simulink model "MSFartoystyring22old"  (Simulink 9.0)
settings: Solver=ode45  StartTime=tstart  StopTime=tstop  RelTol=1e-3  EnableMultiTasking=on
values from neighbouring files (symbols this model uses):
  c = 1    [run22.m]    (also in run23.m = norm(C))
  d1 = -0.0021    [init_controllers.m]
  d2 = 1.0377    [init_controllers.m]
  K = 0.0322    [init_controllers.m]    (also in run_task_1_2.m = x(2))
  Kd = 3*lambda_heading    (= 0.75)    [init_controllers.m]
  Ki = lambda_heading^3    (= 0.015625)    [init_controllers.m]
  Ki_guidance = 0.1    [run22.m]
  Ki_speed = lambda_speed^2    (= 0.09)    [init_controllers.m]
  Kp = 3*lambda_heading^2    (= 0.1875)    [init_controllers.m]
  Kp_guidance = 10    [run22.m]
  Kp_speed = 2*lambda_speed    (= 0.6)    [init_controllers.m]
  m = 5550    [init_controllers.m]
  omega_n = 0.008    [init_controllers.m]
  psi0 = 150*deg2rad    (= 2.61799387799)    [run22.m]    (also in run23.m = 0)
  r0 = 0    [run22.m]    (also in run23.m)
  T = 65.6949    [init_controllers.m]    (also in run_task_1_2.m = 1/x(1))
  tsamp = 10    [run22.m]    (also in run23.m)
  u_r_0 = 100    [init_controllers.m]
  v0 = [6.63 0]'    [run22.m]    (also in run23.m)
undefined symbols (not defined in the file or in its folder): guidance_control, msfartoystyring, WP, zeta
undefined symbols (not defined in the file): p0
settings Model: SuppressorTable=22 serialization::archive 11 0 6 0 0 0 0 0  Creator=christh  LastModifiedBy=henningward  ExtModeAutoUpdateStatusClock=off
settings DataIOCC: LimitDataPoints=on  SignalLoggingSaveFormat=ModelDataLogs
settings OptimizationCC: ExpressionDepthLimit=2147483647  InitFltsAndDblsToZero=on
settings DebuggingCC: SolverPrmCheckMsg=warning  FcnCallInpInsideContextMsg=warning  StateNameClashWarn=warning
settings GRTTargetCC: GeneratePreprocessorConditionals=Disable all  CombineOutputUpdateFcns=off  GRTInterface=on

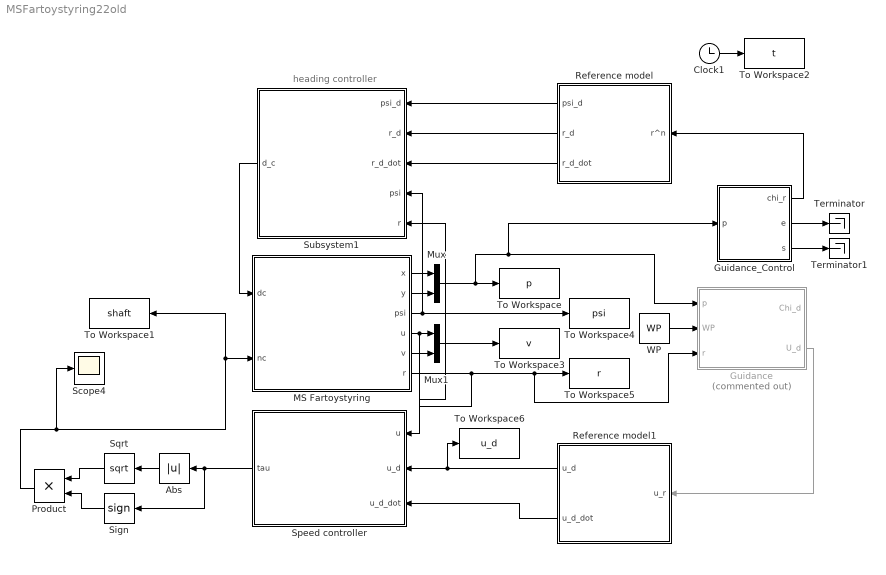
== system MSFartoystyring22old ==
  note: heading controller
  Abs : Abs
  Clock1 : Clock
  "Guidance " : Subsystem  Commented=on
  Guidance_Control : Subsystem
  MS Fartoystyring : Subsystem  mask(MS Fartoystyring for Assignment 3 G&C){x0=p0(1), y0=p0(2), u0=v0(1), v0=v0(2), psi0=psi0, r0=r0, c=c}
      mask prompts: x0 "x(t0) (m)"; y0 "y(t0) (m)"; u0 "u(t0) (m/s)"; v0 "v(t0) (m/s)"; psi0 "psi(t0) (rad)"; r0 "r(t0) (rad/s)"; c "current (0 or 1)"
      mask help:
      | Block corresponding to Figure 1 in the assignment text. Gives the response of the ship.
      |
      | The design speed of MS Fartoystyring is u=8.23 m/s.
      |
      | Input:
      | dc: commanded rudder (rad), dmax=25*pi/180
      | nc: commanded shaft speed (rad/s), nmax=85*2*pi/60
      |
      | Output:
      | x: north pos (m)
      | y: east pos (m)
      | u: surge (m/s)
      | v: sway (m/s)
      | psi: heading (rad)
      | r: yaw (rad/s)
      mask Help: Comments, bugs and help requests can be directed to the TA. Email on course website.
  Mux : Mux  Inputs=2
  Mux1 : Mux  Inputs=2
  Product : Product
  Reference model : Subsystem
  Reference model1 : Subsystem
  Scope4 : Scope
  Sign : Signum
  Speed controller : Subsystem
  Sqrt : Sqrt  SaturateOnIntegerOverflow=on
  Subsystem1 : Subsystem
  Terminator : Terminator
  Terminator1 : Terminator
  To Workspace : ToWorkspace  VariableName=p  SampleTime=tsamp
  To Workspace1 : ToWorkspace  VariableName=shaft  SampleTime=tsamp
  To Workspace2 : ToWorkspace  VariableName=t  SampleTime=tsamp
  To Workspace3 : ToWorkspace  VariableName=v  SampleTime=tsamp
  To Workspace4 : ToWorkspace  VariableName=psi  SampleTime=tsamp
  To Workspace5 : ToWorkspace  VariableName=r  SampleTime=tsamp
  To Workspace6 : ToWorkspace  VariableName=u_d  SampleTime=tsamp
  WP : Constant  Value=WP
  wires:
  MS Fartoystyring/1(x) -> Mux/1
  MS Fartoystyring/2(y) -> Mux/2
  MS Fartoystyring/4(u) -> Speed controller/1("u   "), Mux1/1
  MS Fartoystyring/5(v) -> Mux1/2
  Mux/1 -> Guidance_Control/1(p), "Guidance "/1(p), To Workspace/1
  Mux1/1 -> To Workspace3/1
  MS Fartoystyring/6(r) -> Subsystem1/5(r), "Guidance "/3(r), To Workspace5/1
  Subsystem1/1("d_c ") -> MS Fartoystyring/1(dc)
  Clock1/1 -> To Workspace2/1
  Speed controller/1("tau  ") -> Sign/1, Abs/1
  Abs/1 -> Sqrt/1
  Sign/1 -> Product/2
  Sqrt/1 -> Product/1
  Product/1 -> Scope4/1, To Workspace1/1, MS Fartoystyring/2(nc)
  Reference model/2(r_d) -> Subsystem1/2(r_d)
  Reference model/1(psi_d) -> Subsystem1/1(psi_d)
  Reference model/3(r_d_dot) -> Subsystem1/3(r_d_dot)
  MS Fartoystyring/3(psi) -> To Workspace4/1, Subsystem1/4("psi   ")
  Reference model1/1(u_d) -> To Workspace6/1, Speed controller/2(u_d)
  Reference model1/2(u_d_dot) -> Speed controller/3(u_d_dot)
  "Guidance "/2(U_d) -> Reference model1/1(u_r)
  WP/1 -> "Guidance "/2(WP)
  Guidance_Control/2(e) -> Terminator/1
  Guidance_Control/3(s) -> Terminator1/1
  Guidance_Control/1(chi_r) -> Reference model/1(r^n)

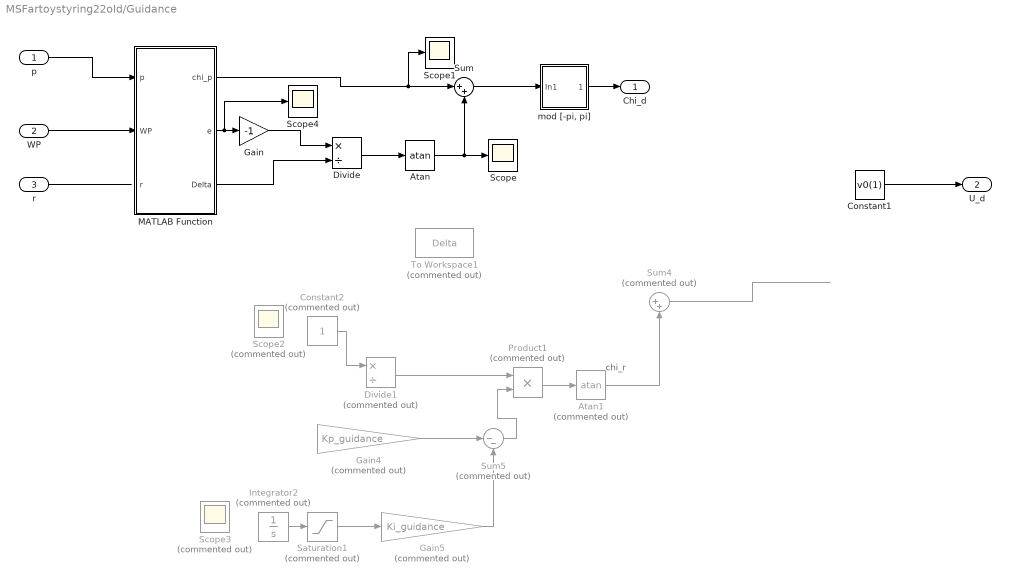
== system MSFartoystyring22old/Guidance  ==
  note: chi_r
  p : Inport
  WP : Inport  Port=2
  r : Inport  Port=3
  Atan : Trigonometry  Operator=atan
  Atan1 : Trigonometry  Commented=on  Operator=atan
  Constant1 : Constant  Value=v0(1)
  Constant2 : Constant  Commented=on
  Divide : Product  Inputs=*/
  Divide1 : Product  Commented=on  Inputs=*/
  Gain : Gain  Gain=-1
  Gain4 : Gain  Commented=on  Gain=Kp_guidance
  Gain5 : Gain  Commented=on  Gain=Ki_guidance
  Integrator2 : Integrator  Commented=on
  MATLAB Function : MATLAB Function  TreatAsAtomicUnit=on
  Product1 : Product  Commented=on
  Saturation1 : Saturate  Commented=on  UpperLimit=inf  LowerLimit=-inf
  Scope : Scope
  Scope1 : Scope
  Scope2 : Scope  Commented=on
  Scope3 : Scope  Commented=on
  Scope4 : Scope
  Sum : Sum  Inputs=|++
  Sum4 : Sum  Commented=on  Inputs=|++
  Sum5 : Sum  Commented=on  Inputs=|--
  To Workspace1 : ToWorkspace  Commented=on  VariableName=Delta  SampleTime=-1
  "mod [-pi, pi]" : Subsystem
  "Chi_d " : Outport
  U_d : Outport  Port=2
  wires:
  p/1 -> MATLAB Function/1(p)
  WP/1 -> MATLAB Function/2(WP)
  r/1 -> ?
  Constant1/1 -> U_d/1
  Sum4/1 -> ?
  Gain5/1 -> Sum5/2
  Sum5/1 -> Product1/2
  Integrator2/1 -> Saturation1/1
  Atan1/1 -> Sum4/2
  ? -> Scope3/1, To Workspace1/1, Divide1/2
  ? -> Integrator2/1, Gain4/1, Scope2/1
  Divide1/1 -> Product1/1
  Gain4/1 -> Sum5/1
  Constant2/1 -> Divide1/1
  Product1/1 -> Atan1/1
  Saturation1/1 -> Gain5/1
  ? -> Sum4/1
  MATLAB Function/3(Delta) -> Divide/2
  MATLAB Function/2(e) -> Scope4/1, Gain/1
  Gain/1 -> Divide/1
  Divide/1 -> Atan/1
  MATLAB Function/1(chi_p) -> Scope1/1, Sum/1
  Atan/1 -> Scope/1, Sum/2
  Sum/1 -> "mod [-pi, pi]"/1(In1)
  "mod [-pi, pi]"/1(Out1) -> "Chi_d "/1

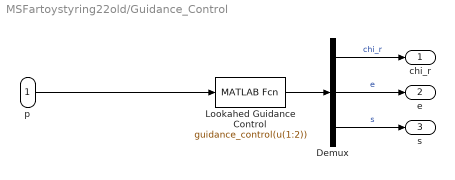
== system MSFartoystyring22old/Guidance_Control ==
  p : Inport
  Demux : Demux  Outputs=3
  Lookahed Guidance Control : MATLABFcn  MATLABFcn=guidance_control(u(1:2))  OutputDimensions=3
  chi_r : Outport
  e : Outport  Port=2
  s : Outport  Port=3
  wires:
  Lookahed Guidance Control/1 -> Demux/1
  Demux/2 -> e/1  "e"
  Demux/1 -> chi_r/1  "chi_r"
  Demux/3 -> s/1  "s"
  p/1 -> Lookahed Guidance Control/1

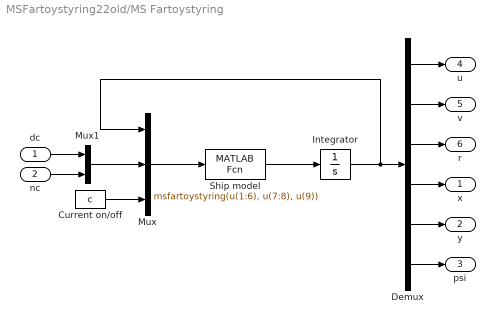
== system MSFartoystyring22old/MS Fartoystyring ==
  dc : Inport
  nc : Inport  Port=2
  Current on/off : Constant  Value=c
  Demux : Demux  Outputs=6
  Integrator : Integrator  InitialCondition=[u0 v0 r0 x0 y0 psi0]'
  Mux : Mux  Inputs=3
  Mux1 : Mux  Inputs=2
  Ship model : MATLABFcn  MATLABFcn=msfartoystyring(u(1:6), u(7:8), u(9))  OutputDimensions=6
  x : Outport
  y : Outport  Port=2
  psi : Outport  Port=3
  u : Outport  Port=4
  v : Outport  Port=5
  r : Outport  Port=6
  wires:
  Integrator/1 -> Mux/1, Demux/1
  Mux1/1 -> Mux/2
  dc/1 -> Mux1/1
  nc/1 -> Mux1/2
  Demux/1 -> u/1
  Demux/2 -> v/1
  Demux/3 -> r/1
  Demux/4 -> x/1
  Demux/5 -> y/1
  Demux/6 -> psi/1
  Current on/off/1 -> Mux/3
  Ship model/1 -> Integrator/1
  Mux/1 -> Ship model/1

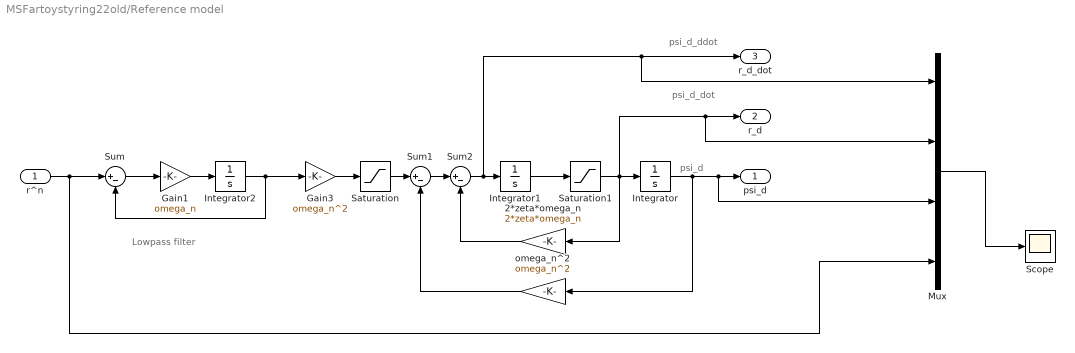
== system MSFartoystyring22old/Reference model ==
  note: psi_d_ddot
  note: psi_d_dot
  note: Lowpass filter
  note: psi_d
  r^n : Inport
  2*zeta*omega_n : Gain  Gain=2*zeta*omega_n
  Gain1 : Gain  Gain=omega_n
  Gain3 : Gain  Gain=omega_n^2
  Integrator : Integrator
  Integrator1 : Integrator
  Integrator2 : Integrator
  Mux : Mux
  Saturation : Saturate  UpperLimit=1000  LowerLimit=-1000
  Saturation1 : Saturate  UpperLimit=1000  LowerLimit=-1000
  Scope : Scope
  Sum : Sum  Inputs=|+-
  Sum1 : Sum  Inputs=|+-
  Sum2 : Sum  Inputs=|+-
  omega_n^2 : Gain  Gain=omega_n^2
  psi_d : Outport
  r_d : Outport  Port=2
  r_d_dot : Outport  Port=3
  wires:
  Integrator1/1 -> Saturation1/1
  Saturation1/1 -> Mux/2, r_d/1, 2*zeta*omega_n/1, Integrator/1
  2*zeta*omega_n/1 -> Sum2/2
  Sum2/1 -> Mux/1, r_d_dot/1, Integrator1/1
  omega_n^2/1 -> Sum1/2
  Saturation/1 -> Sum1/1
  Gain3/1 -> Saturation/1
  Sum1/1 -> Sum2/1
  Sum/1 -> Gain1/1
  Integrator2/1 -> Sum/2, Gain3/1
  Gain1/1 -> Integrator2/1
  Integrator/1 -> Mux/3, psi_d/1, omega_n^2/1
  r^n/1 -> Mux/4, Sum/1
  Mux/1 -> Scope/1

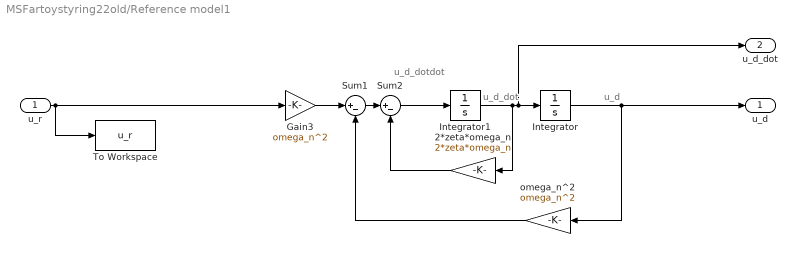
== system MSFartoystyring22old/Reference model1 ==
  note: u_d
  note: u_d_dot
  note: u_d_dotdot
  u_r : Inport
  2*zeta*omega_n : Gain  Gain=2*zeta*omega_n
  Gain3 : Gain  Gain=omega_n^2
  Integrator : Integrator  InitialCondition=u_r_0
  Integrator1 : Integrator
  Sum1 : Sum  Inputs=|+-
  Sum2 : Sum  Inputs=|+-
  To Workspace : ToWorkspace  VariableName=u_r  SampleTime=-1
  omega_n^2 : Gain  Gain=omega_n^2
  u_d : Outport
  u_d_dot : Outport  Port=2
  wires:
  Integrator1/1 -> 2*zeta*omega_n/1, Integrator/1, u_d_dot/1
  2*zeta*omega_n/1 -> Sum2/2
  Sum1/1 -> Sum2/1
  omega_n^2/1 -> Sum1/2
  Gain3/1 -> Sum1/1
  Sum2/1 -> Integrator1/1
  Integrator/1 -> omega_n^2/1, u_d/1
  u_r/1 -> To Workspace/1, Gain3/1

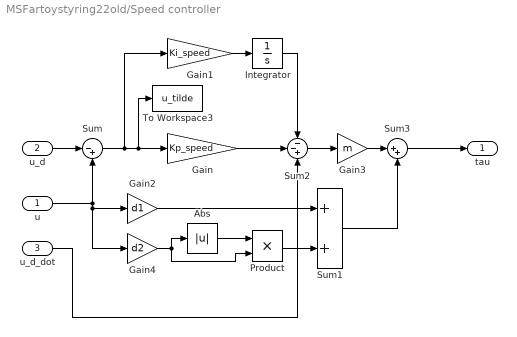
== system MSFartoystyring22old/Speed controller ==
  "u   " : Inport
  u_d : Inport  Port=2
  u_d_dot : Inport  Port=3
  Abs : Abs
  Gain : Gain  Gain=Kp_speed
  Gain1 : Gain  Gain=Ki_speed
  Gain2 : Gain  Gain=d1
  Gain3 : Gain  Gain=m
  Gain4 : Gain  Gain=d2
  Integrator : Integrator
  Product : Product
  Sum : Sum  Inputs=|-+
  Sum1 : Sum
  Sum2 : Sum  Inputs=--+
  Sum3 : Sum  Inputs=|++
  To Workspace3 : ToWorkspace  VariableName=u_tilde  SampleTime=tsamp
  "tau  " : Outport
  wires:
  Integrator/1 -> Sum2/1
  Gain/1 -> Sum2/2
  Sum2/1 -> Gain3/1
  Gain3/1 -> Sum3/1
  u_d_dot/1 -> Sum2/3
  Sum/1 -> To Workspace3/1, Gain/1, Gain1/1
  Gain1/1 -> Integrator/1
  u_d/1 -> Sum/1
  "u   "/1 -> Gain4/1, Gain2/1, Sum/2
  Abs/1 -> Product/1
  Gain4/1 -> Abs/1, Product/2
  Gain2/1 -> Sum1/1
  Product/1 -> Sum1/2
  Sum1/1 -> Sum3/2
  Sum3/1 -> "tau  "/1

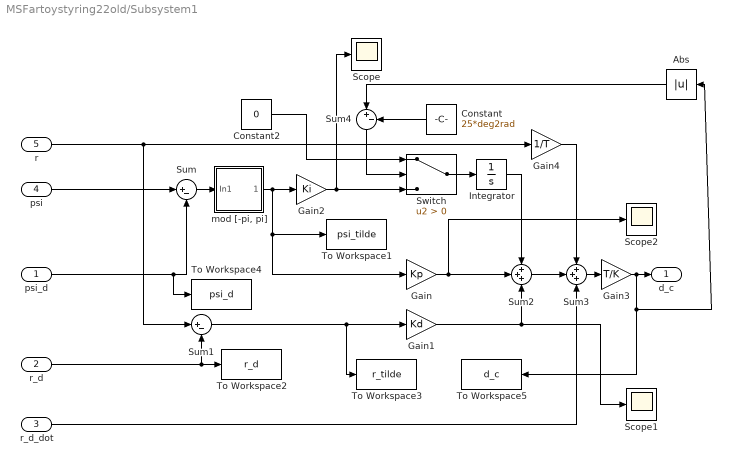
== system MSFartoystyring22old/Subsystem1 ==
  psi_d : Inport
  r_d : Inport  Port=2
  r_d_dot : Inport  Port=3
  "psi   " : Inport  Port=4
  r : Inport  Port=5
  Abs : Abs
  Constant : Constant  Value=25*deg2rad
  Constant2 : Constant  Value=0
  Gain : Gain  Gain=Kp
  Gain1 : Gain  Gain=Kd
  Gain2 : Gain  Gain=Ki
  Gain3 : Gain  Gain=T/K
  Gain4 : Gain  Gain=1/T
  Integrator : Integrator  LimitOutput=on  UpperSaturationLimit=deg2rad*25  LowerSaturationLimit=-deg2rad*26
  Scope : Scope
  Scope1 : Scope
  Scope2 : Scope
  Sum : Sum  Inputs=|+-
  Sum1 : Sum  Inputs=|+-
  Sum2 : Sum  Inputs=+++
  Sum3 : Sum  Inputs=+++
  Sum4 : Sum  Inputs=|+-
  Switch : Switch  Criteria=u2 > Threshold
  To Workspace1 : ToWorkspace  VariableName=psi_tilde  SampleTime=tsamp
  To Workspace2 : ToWorkspace  VariableName=r_d  SampleTime=tsamp
  To Workspace3 : ToWorkspace  VariableName=r_tilde  SampleTime=tsamp
  To Workspace4 : ToWorkspace  VariableName=psi_d  SampleTime=tsamp
  To Workspace5 : ToWorkspace  VariableName=d_c  SampleTime=tsamp
  "mod [-pi, pi]" : Subsystem
  "d_c " : Outport
  wires:
  "psi   "/1 -> Sum/1
  r_d/1 -> To Workspace2/1, Sum1/2
  Sum1/1 -> To Workspace3/1, Gain1/1
  Integrator/1 -> Sum2/1
  Sum/1 -> "mod [-pi, pi]"/1(In1)
  Gain2/1 -> Switch/3, Scope/1
  Gain/1 -> Scope2/1, Sum2/2
  Gain1/1 -> Scope1/1, Sum2/3
  psi_d/1 -> To Workspace4/1, Sum/2
  Switch/1 -> Integrator/1
  Gain3/1 -> To Workspace5/1, Abs/1, "d_c "/1
  Sum3/1 -> Gain3/1
  Sum2/1 -> Sum3/2
  r/1 -> Sum1/1, Gain4/1
  Abs/1 -> Sum4/1
  Constant/1 -> Sum4/2
  Sum4/1 -> Switch/2
  Constant2/1 -> Switch/1
  Gain4/1 -> Sum3/1
  r_d_dot/1 -> Sum3/3
  "mod [-pi, pi]"/1(Out1) -> Gain/1, To Workspace1/1, Gain2/1

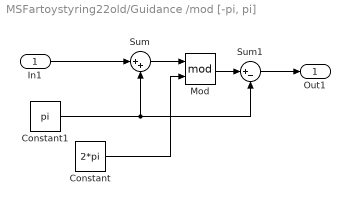
== system MSFartoystyring22old/Guidance /mod [-pi, pi] ==
  In1 : Inport
  Constant : Constant  Value=2*pi
  Constant1 : Constant  Value=pi
  Mod : Math  Operator=mod  SaturateOnIntegerOverflow=on
  Sum : Sum  Inputs=|++
  Sum1 : Sum  Inputs=|+-
  Out1 : Outport
  wires:
  Constant/1 -> Mod/2
  In1/1 -> Sum/1
  Constant1/1 -> Sum1/2, Sum/2
  Sum/1 -> Mod/1
  Mod/1 -> Sum1/1
  Sum1/1 -> Out1/1

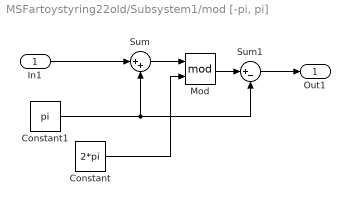
== system MSFartoystyring22old/Subsystem1/mod [-pi, pi] ==
  In1 : Inport
  Constant : Constant  Value=2*pi
  Constant1 : Constant  Value=pi
  Mod : Math  Operator=mod  SaturateOnIntegerOverflow=on
  Sum : Sum  Inputs=|++
  Sum1 : Sum  Inputs=|+-
  Out1 : Outport
  wires:
  Constant/1 -> Mod/2
  In1/1 -> Sum/1
  Constant1/1 -> Sum1/2, Sum/2
  Sum/1 -> Mod/1
  Mod/1 -> Sum1/1
  Sum1/1 -> Out1/1

== matlab function Guidance /MATLAB Function ==
  settings: updateMethod=DISCRETE  sampleTime=tsamp
  data: p input double; chi_p output double; WP input double; e output double; Delta output double; r input double
function [chi_p, e, Delta] = fcn(p, WP, r)
    
    %number of waypoints
    N = length(WP);
    
    % waypoint iteration
    persistent k;
    
    
    
    %current position
    x_current = p(1);
    y_current = p(2);
    
    %waypoint iteration
    if (isempty(k))
        k = 2;
    end
    %current waypoint
    xk_1 = WP(1, k-1);
    yk_1 = WP(2, k-1);
    
    %next waypoint
    xk_2 = WP(1, k);
    yk_2 = WP(2, k);
    
    %{
    if k ~= 6 && k ~= 1
        %calculating optimal turningradius
        lastWP = [WP(1,k-1); WP(2,k-1)];
        currentWP = [WP(1,k); WP(2,k)]; %way points
        nextWP = [WP(1,k+1); WP(2,k+1)];
        u = (lastWP - currentWP)/(norm(lastWP-currentWP));
        v = (nextWP - currentWP)/(norm(nextWP-currentWP)); %a,b,c
        w = (u + v)/(norm(u + v));
        a = acos((norm(v)^2 + norm(u+v)^2 - norm(u)^2)/(2*norm(v)*norm(u+v)));
        turningRadius = 365 / sin(a) * 1.2;
    else
        turningRadius = 365;
    end
    %}
   
    
    
    
    
    alpha = atan2(yk_2-yk_1, xk_2-xk_1);
    
    Rp = [cos(alpha) -sin(alpha);
          sin(alpha) cos(alpha);];
    
    epsilon = Rp'*([x_current y_current]' - [xk_1 yk_1]');
    
    %R = sqrt(((xk_2-xk_1)^2+(yk_2-yk_1)^2))-epsilon(1,:); %Radius of acceptance
    chi_p = alpha;
    e = epsilon(2);
    
    if ((((xk_1 - x_current)^2 + (yk_1 - y_current)^2) <= 900^2) && (N > k))
        k = k + 1;
    end   
    
    
    Delta = 600;
    
end
